simulink model "betalink_test"  (R2020b)
settings: Solver=FixedStepDiscrete  StartTime=0.0  StopTime=Inf  RelTol=1e-3
libraries: simulink x8, rpi_blkst x2
settings Model: SimulationMode=external  Creator=jacques  LastModifiedBy=jacques
settings DataIOCC: ReturnWorkspaceOutputs=off
settings OptimizationCC: EnhancedBackFolding=on  PassReuseOutputArgsAs=Individual arguments  ZeroExternalMemoryAtStartup=off  ZeroInternalMemoryAtStartup=off  OptimizeBlockOrder=speed  DifferentSizesBufferReuse=on  OptimizationCustomize=off  EfficientTunableParamExpr=on
settings DebuggingCC: ParameterTunabilityLossMsg=error
settings HardwareCC: ProdBitPerLong=64  ProdLargestAtomicInteger=LongLong  ProdLargestAtomicFloat=Double  ProdLongLongMode=on  ProdHWDeviceType=ARM Compatible->ARM 64-bit (LP64)
settings SFSimCC: MATLABDynamicMemAlloc=off
settings RTWCC: Description=RTW Embedded Coder RPI target  SystemTargetFile=ert_rpi.tlc  TemplateMakefile=ert_rpi.tmf  PostCodeGenCommand=postGenFunc(buildInfo)
settings CodeAppCC: ForceParamTrailComments=on  IgnoreCustomStorageClasses=off  OperatorAnnotations=on  SimulinkDataObjDesc=on  SFDataObjDesc=on  InsertBlockDesc=on
settings STFCustomTargetCC: TargetLangStandard=C99 (ISO)  MultiwordLength=256  ModelReferenceCompliant=off  ConcurrentExecutionCompliant=off  CombineOutputUpdateFcns=on  ERTCustomFileBanners=on  SupportNonInlinedSFcns=off  RemoveResetFunc=on  MATLABClassNameForMDSCustomization=Simulink.SoftwareTarget.ERTCustomization  CPPClassGenCompliant=off  GRTInterface=off  SystemTargetFile=ert_rpi.tlc
settings ERTTargetCC: TargetLangStandard=C99 (ISO)  ModelReferenceCompliant=off  ParMdlRefBuildCompliant=off  CompOptLevelCompliant=off  ConcurrentExecutionCompliant=off  SupportContinuousTime=on  ModelStepFunctionPrototypeControlCompliant=off  CPPClassGenCompliant=off  UseToolchainInfoCompliant=off  ExtMode=on  ExtModeMexArgs='192.168.132.154'  ERTCustomFileTemplate=ert_rpi_file_process.tlc

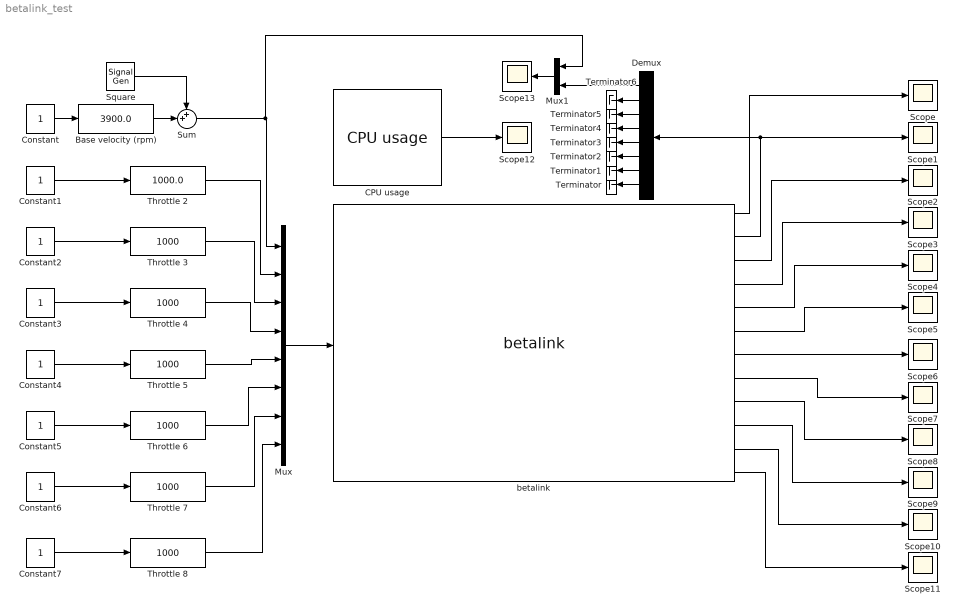
== system betalink_test ==
  Base velocity (rpm) : simulink/Math Operations/Slider Gain  gain=3900.0  low=2500  high=20000
  CPU usage : rpi_blkst/CPU usage  rpi_mask_Ts=0.004
      settings: SourceProductName=RPI Blockset
  Constant{,1..7} (8 alike) : Constant  SampleTime=-1
  Demux : Demux  Outputs=8
  Mux : Mux  Inputs=8
  Mux1 : Mux  Inputs=2
  Scope{,1..13} (14 alike) : Scope
  Square : SignalGenerator  WaveForm=square  Amplitude=200
  Sum : Sum  Inputs=++|
  Terminator{,1..6} (7 alike) : Terminator
  Throttle 2 : simulink/Math Operations/Slider Gain  gain=1000.0  low=1000  high=1400
  Throttle {3..8} (6 alike) : simulink/Math Operations/Slider Gain  gain=1000  low=1000  high=1400
  betalink : rpi_blkst/betalink  rpi_mask_usb_serial_number=643986269  rpi_mask_Ts=0.004
      settings: SourceProductName=RPI Blockset
  wires:
  Constant/1 -> Base velocity (rpm)/1
  betalink/1 -> Scope/1
  betalink/2 -> Demux/1, Scope1/1
  betalink/3 -> Scope2/1
  betalink/4 -> Scope3/1
  betalink/5 -> Scope4/1
  betalink/6 -> Scope5/1
  betalink/7 -> Scope6/1
  betalink/8 -> Scope7/1
  betalink/9 -> Scope8/1
  betalink/10 -> Scope9/1
  betalink/11 -> Scope10/1
  betalink/12 -> Scope11/1
  Constant1/1 -> Throttle 2/1
  Constant2/1 -> Throttle 3/1
  Constant3/1 -> Throttle 4/1
  Constant4/1 -> Throttle 5/1
  Constant5/1 -> Throttle 6/1
  Constant6/1 -> Throttle 7/1
  Constant7/1 -> Throttle 8/1
  Mux/1 -> betalink/1
  Throttle 2/1 -> Mux/2
  Throttle 3/1 -> Mux/3
  Throttle 4/1 -> Mux/4
  Throttle 5/1 -> Mux/5
  Throttle 6/1 -> Mux/6
  Throttle 7/1 -> Mux/7
  Throttle 8/1 -> Mux/8
  CPU usage/1 -> Scope12/1
  Base velocity (rpm)/1 -> Sum/2
  Sum/1 -> Mux1/1, Mux/1
  Square/1 -> Sum/1
  Demux/7 -> Terminator1/1
  Demux/6 -> Terminator2/1
  Demux/8 -> Terminator/1
  Demux/5 -> Terminator3/1
  Demux/4 -> Terminator4/1
  Demux/3 -> Terminator5/1
  Demux/2 -> Terminator6/1
  Mux1/1 -> Scope13/1
  Demux/1 -> Mux1/2
